simulink model "config5sim_KinematicController_generator"  (R2019b)
settings: Solver=ode4  StartTime=0.0  StopTime=80  FixedStep=0.025  RelTol=1e-3  EnableMultiTasking=on
InitFcn:
  | if set_path == 1
  |     Ref_Path1;
  | elseif set_path == 2
  |     Ref_Path2;
  | elseif set_path == 3
  |     Ref_Path3;
  | end
  | 
  | roboparam;
StopFcn:
  | figure(double(set_path))
  | plot(xyref.DATA(:,1),xyref.DATA(:,2),'--black')
  | hold on
  | plot(xy_axon.DATA(:,1),xy_axon.DATA(:,2),'red')
  | hold on
  | plot(xy_trolley.DATA(:,1),xy_trolley.DATA(:,2),'green')
  | hold on
  | legend('Reference trajectory', 'Robot trajectory', 'Trailer trajectory')
values from neighbouring files (symbols this model uses):
  L = 0.387/2    (= 0.1935)    [AXON_Dynamics_CONF5_vw_old.m]    (also in roboparam.m)
  psicw10 = 0    [roboparam.m]
  psicw20 = 0    [roboparam.m]
  psicw30 = 0    [roboparam.m]
  psicw40 = 0    [roboparam.m]
  rho0 = 0.5    [AXON_Dynamics_CONF5_vw_old.m]    (also in roboparam.m)
  rho1 = 1    [AXON_Dynamics_CONF5_vw_old.m]    (also in roboparam.m)
  rhoH = 0.075    [AXON_Dynamics_CONF5_vw_old.m]    (also in roboparam.m)
  th0 = z(4)    [AXON_Dynamics_CONF5_vw_old.m]    (also in AllInOneDynamic.m = th(i,2); Kinematics.m; PathGenerationPlotting_Dynamics.m = th(i,2); PathGenerationPlotting_Kinematics.m = z(i,4))
  th1 = z(3)    [AXON_Dynamics_CONF5_vw_old.m]    (also in AllInOneDynamic.m = th(i,1); Kinematics.m; PathGenerationPlotting_Dynamics.m = th(i,1); PathGenerationPlotting_Kinematics.m = z(i,3))
  v0 = 0    [roboparam.m]
  w0 = 0    [roboparam.m]
  xaxon0 = xtrolley0+rho1*cos(th1)+rho0*cos(th0)    [roboparam.m]
  xtrolley0 = 0    [roboparam.m]
  yaxon0 = ytrolley0+rho1*sin(th1)+rho0*sin(th0)    [roboparam.m]
  ytrolley0 = 0    [roboparam.m]
undefined symbols (not defined in the file or in its folder): sigbuilder_block
libraries: simulink x2
settings Model: Creator=e0010448  LastModifiedBy=vladkhon
settings DataIOCC: LimitDataPoints=on  SaveFormat=StructureWithTime  ReturnWorkspaceOutputs=off
settings OptimizationCC: BlockReduction=off  BufferReuse=off  LifeSpan=inf
settings DebuggingCC: AlgebraicLoopMsg=none  UnconnectedInputMsg=none  UnconnectedOutputMsg=none  UnconnectedLineMsg=none  AllowSymbolicDim=off  SFUnexpectedBacktrackingDiag=warning  SFNoUnconditionalDefaultTransitionDiag=warning  SFExecutionAtInitializationDiag=none  ArithmeticOperatorsInVariantConditions=warning
settings HardwareCC: ProdBitPerPointer=32  ProdBitPerSizeT=32  ProdBitPerPtrDiffT=32  ProdLargestAtomicFloat=None  ProdIntDivRoundTo=Undefined  ProdEndianess=Unspecified  ProdWordSize=32  ProdHWDeviceType=32-bit Generic
settings ModelReferenceCC: PropagateSignalLabelsOutOfModel=off
settings SFSimCC: SimUseLocalCustomCode=off  CustomCodeUndefinedFunction=UseInterfaceOnly
settings RTWCC: RTWUseLocalCustomCode=off
settings CodeAppCC: StateflowObjectComments=on
settings GRTTargetCC: TargetLangStandard=C89/C90 (ANSI)  GeneratePreprocessorConditionals=Disable all
settings ConfigComp: CovMetricSettings=dw  CovHtmlReporting=on  CovSaveCumulativeToWorkspaceVar=on  CovSaveSingleToWorkspaceVar=on  CovExternalEMLEnable=off

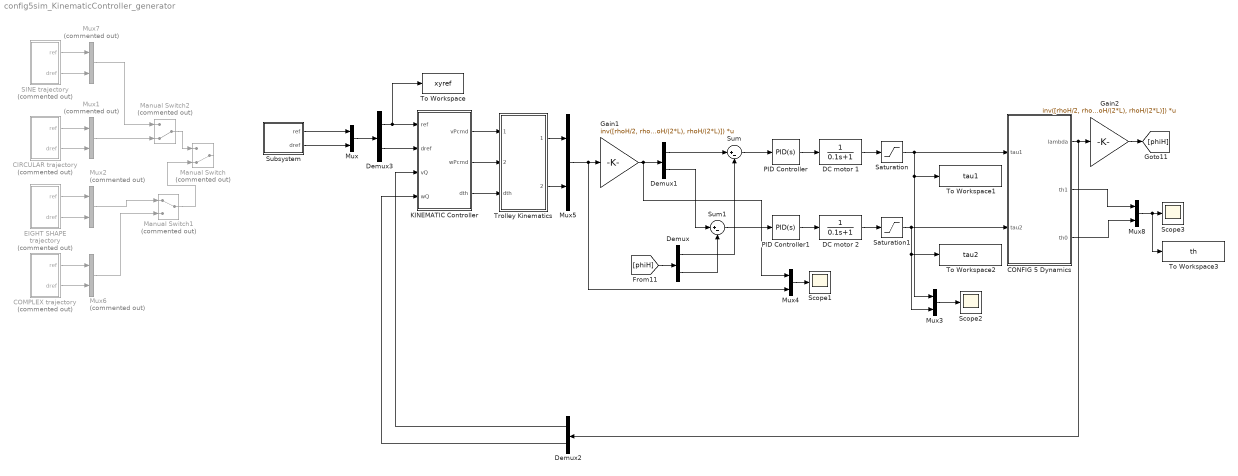
== system config5sim_KinematicController_generator ==
  CIRCULAR trajectory : Subsystem  Commented=on
  COMPLEX trajectory : Subsystem  Commented=on
  CONFIG 5 Dynamics : Subsystem
  DC motor 1 : TransferFcn  Denominator=[0.1 1]
  DC motor 2 : TransferFcn  Denominator=[0.1 1]
  Demux{,1..3} (4 alike) : Demux  Outputs=2
  EIGHT SHAPE trajectory : Subsystem  Commented=on
  Gain1 : Gain  Gain=inv([rhoH/2, rhoH/2; -rhoH/(2*L), rhoH/(2*L)])  Multiplication=Matrix(K*u)
  Gain2 : Gain  Gain=inv([rhoH/2, rhoH/2; -rhoH/(2*L), rhoH/(2*L)])  Multiplication=Matrix(K*u)
  KINEMATIC Controller : Subsystem
  Manual Switch : ManualSwitch  Commented=on  CurrentSetting=0
  Manual Switch1 : ManualSwitch  Commented=on
  Manual Switch2 : ManualSwitch  Commented=on  CurrentSetting=0
  Mux{,3..5,8} (5 alike) : Mux  Inputs=2
  Mux{1..2,6..7} (4 alike) : Mux  Commented=on  Inputs=2
  PID Controller : simulink/Continuous/PID Controller  Controller=PID  Form=Parallel  TimeDomain=Continuous-time  SampleTime=-1  IntegratorMethod=Forward Euler  FilterMethod=Forward Euler  ControllerParametersSource=internal  P=3  I=5  D=1  UseFilter=on  N=100  TunerSelectOption=Transfer Function Based (PID Tuner App)  InitialConditionSource=internal  InitialConditionForIntegrator=0  InitialConditionForFilter=0  DifferentiatorICPrevScaledInput=0  ExternalReset=none  TrackingMode=off  Kt=1  LimitOutput=off  UpperSaturationLimit=inf  LowerSaturationLimit=-inf  LinearizeAsGain=on  AntiWindupMode=none  Kb=1  POutMin=[]  POutMax=[]  IOutMin=[]  IOutMax=[]  DOutMin=[]  DOutMax=[]  NOutMin=[]  NOutMax=[]  SumOutMin=[]  SumOutMax=[]  SaturationOutMin=[]  SaturationOutMax=[]  PParamMin=[]  PParamMax=[]  IParamMin=[]  IParamMax=[]  DParamMin=[]  DParamMax=[]  NParamMin=[]  NParamMax=[]  KbParamMin=[]  KbParamMax=[]  KtParamMin=[]  KtParamMax=[]  KbOutMin=[]  KbOutMax=[]  KtOutMin=[]  KtOutMax=[]  IntegratorOutMin=[]  IntegratorOutMax=[]  FilterOutMin=[]  FilterOutMax=[]  SumI1OutMin=[]  SumI1OutMax=[]  SumI2OutMin=[]  SumI2OutMax=[]  SumI3OutMin=[]  SumI3OutMax=[]  SumI4OutMin=[]  SumI4OutMax=[]  SumDOutMin=[]  SumDOutMax=[]  DifferentiatorOutMin=[]  DifferentiatorOutMax=[]  FilterDiffOutCoefMin=[]  FilterDiffOutCoefMax=[]  ReciprocalOutMin=[]  ReciprocalOutMax=[]  SumDenOutMin=[]  SumDenOutMax=[]  SumNumOutMin=[]  SumNumOutMax=[]  DivideOutMin=[]  DivideOutMax=[]  IntegratorContinuousStateAttributes=''  IntegratorStateMustResolveToSignalObject=off  IntegratorRTWStateStorageClass=Auto  FilterContinuousStateAttributes=''  FilterStateMustResolveToSignalObject=off  FilterRTWStateStorageClass=Auto  ParallelPVariant=InternalParameters  IdealPVariant=Disabled  IVariant=InternalParameters  DVariant=InternalParameters  IntegratorVariant=Continuous  SatVariant=Disabled  AWVariant=Passthrough  PCopyVariant=Disabled  TRVariant=Disabled  FdbkBlocksVariant=Forward  IdealPFdbkVariant=Disabled  SatFdbkVariant=Disabled  DerivativeFilterVariant=ContFilter  NVariant=InternalParameters  NCopyVariant=Disabled  FilterICVariant=InternalICsFilter  IntegratorICVariant=InternalICs  ExternalResetVariant=Disabled  TRSumVariant=Passthrough  SumFdbkVariant=Disabled  SumVariant=Sum_PID
  PID Controller1 : simulink/Continuous/PID Controller  Controller=PID  Form=Parallel  TimeDomain=Continuous-time  SampleTime=-1  IntegratorMethod=Forward Euler  FilterMethod=Forward Euler  ControllerParametersSource=internal  P=3  I=5  D=1  UseFilter=on  N=100  TunerSelectOption=Transfer Function Based (PID Tuner App)  InitialConditionSource=internal  InitialConditionForIntegrator=0  InitialConditionForFilter=0  DifferentiatorICPrevScaledInput=0  ExternalReset=none  TrackingMode=off  Kt=1  LimitOutput=off  UpperSaturationLimit=inf  LowerSaturationLimit=-inf  LinearizeAsGain=on  AntiWindupMode=none  Kb=1  POutMin=[]  POutMax=[]  IOutMin=[]  IOutMax=[]  DOutMin=[]  DOutMax=[]  NOutMin=[]  NOutMax=[]  SumOutMin=[]  SumOutMax=[]  SaturationOutMin=[]  SaturationOutMax=[]  PParamMin=[]  PParamMax=[]  IParamMin=[]  IParamMax=[]  DParamMin=[]  DParamMax=[]  NParamMin=[]  NParamMax=[]  KbParamMin=[]  KbParamMax=[]  KtParamMin=[]  KtParamMax=[]  KbOutMin=[]  KbOutMax=[]  KtOutMin=[]  KtOutMax=[]  IntegratorOutMin=[]  IntegratorOutMax=[]  FilterOutMin=[]  FilterOutMax=[]  SumI1OutMin=[]  SumI1OutMax=[]  SumI2OutMin=[]  SumI2OutMax=[]  SumI3OutMin=[]  SumI3OutMax=[]  SumI4OutMin=[]  SumI4OutMax=[]  SumDOutMin=[]  SumDOutMax=[]  DifferentiatorOutMin=[]  DifferentiatorOutMax=[]  FilterDiffOutCoefMin=[]  FilterDiffOutCoefMax=[]  ReciprocalOutMin=[]  ReciprocalOutMax=[]  SumDenOutMin=[]  SumDenOutMax=[]  SumNumOutMin=[]  SumNumOutMax=[]  DivideOutMin=[]  DivideOutMax=[]  IntegratorContinuousStateAttributes=''  IntegratorStateMustResolveToSignalObject=off  IntegratorRTWStateStorageClass=Auto  FilterContinuousStateAttributes=''  FilterStateMustResolveToSignalObject=off  FilterRTWStateStorageClass=Auto  ParallelPVariant=InternalParameters  IdealPVariant=Disabled  IVariant=InternalParameters  DVariant=InternalParameters  IntegratorVariant=Continuous  SatVariant=Disabled  AWVariant=Passthrough  PCopyVariant=Disabled  TRVariant=Disabled  FdbkBlocksVariant=Forward  IdealPFdbkVariant=Disabled  SatFdbkVariant=Disabled  DerivativeFilterVariant=ContFilter  NVariant=InternalParameters  NCopyVariant=Disabled  FilterICVariant=InternalICsFilter  IntegratorICVariant=InternalICs  ExternalResetVariant=Disabled  TRSumVariant=Passthrough  SumFdbkVariant=Disabled  SumVariant=Sum_PID
  SINE trajectory : Subsystem  Commented=on
  Saturation : Saturate  UpperLimit=40  LowerLimit=-40
  Saturation1 : Saturate  UpperLimit=40  LowerLimit=-40
  Scope1 : Scope
  Scope2 : Scope
  Scope3 : Scope
  Subsystem : Subsystem
  Sum : Sum  Inputs=|+-
  Sum1 : Sum  Inputs=|+-
  To Workspace : ToWorkspace  VariableName=xyref  SaveFormat=Timeseries  SampleTime=-1
  To Workspace1 : ToWorkspace  VariableName=tau1  SampleTime=-1
  To Workspace2 : ToWorkspace  VariableName=tau2  SampleTime=-1
  To Workspace3 : ToWorkspace  VariableName=th  SampleTime=-1
  Trolley Kinematics : Subsystem
  wires:
  Sum/1 -> PID Controller/1
  CONFIG 5 Dynamics/1(lambda) -> Gain2/1, Demux2/1
  [phiH] -> Demux/1
  Demux/1 -> Sum/2
  Demux/2 -> Sum1/2
  Sum1/1 -> PID Controller1/1
  Mux4/1 -> Scope1/1
  Mux5/1 -> Mux4/2, Gain1/1
  Gain2/1 -> [phiH]
  Demux1/1 -> Sum/1
  Demux1/2 -> Sum1/1
  Mux3/1 -> Scope2/1
  Gain1/1 -> Mux4/1, Demux1/1
  PID Controller/1 -> DC motor 1/1
  PID Controller1/1 -> DC motor 2/1
  Demux2/1 -> KINEMATIC Controller/3(vQ)
  Demux2/2 -> KINEMATIC Controller/4(wQ)
  CIRCULAR trajectory/1(ref) -> Mux1/1
  CIRCULAR trajectory/2(dref) -> Mux1/2
  Demux3/1 -> To Workspace/1, KINEMATIC Controller/1(ref)
  Demux3/2 -> KINEMATIC Controller/2(dref)
  EIGHT SHAPE trajectory/1(ref) -> Mux2/1
  EIGHT SHAPE trajectory/2(dref) -> Mux2/2
  Mux2/1 -> Manual Switch1/1
  Manual Switch1/1 -> Manual Switch/2
  Mux6/1 -> Manual Switch1/2
  COMPLEX trajectory/1(ref) -> Mux6/1
  COMPLEX trajectory/2(dref) -> Mux6/2
  Manual Switch2/1 -> Manual Switch/1
  Mux1/1 -> Manual Switch2/2
  Mux7/1 -> Manual Switch2/1
  SINE trajectory/1(ref) -> Mux7/1
  SINE trajectory/2(dref) -> Mux7/2
  DC motor 1/1 -> Saturation/1
  Saturation/1 -> To Workspace1/1, Mux3/1, CONFIG 5 Dynamics/1(tau1)
  DC motor 2/1 -> Saturation1/1
  Saturation1/1 -> To Workspace2/1, Mux3/2, CONFIG 5 Dynamics/2(tau2)
  KINEMATIC Controller/1(vPcmd) -> Trolley Kinematics/1(vPcmd)
  KINEMATIC Controller/2(wPcmd) -> Trolley Kinematics/2(wPcmd)
  Trolley Kinematics/1(vQcmd) -> Mux5/1
  Trolley Kinematics/2(wQcmd) -> Mux5/2
  KINEMATIC Controller/3(dth) -> Trolley Kinematics/3(dth)
  Mux8/1 -> To Workspace3/1, Scope3/1
  Subsystem/2("dref ") -> Mux/2
  Subsystem/1(ref) -> Mux/1
  Mux/1 -> Demux3/1
  CONFIG 5 Dynamics/3(th0) -> Mux8/2
  CONFIG 5 Dynamics/2(th1) -> Mux8/1

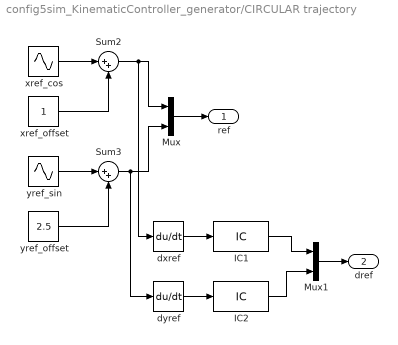
== system config5sim_KinematicController_generator/CIRCULAR trajectory ==
  IC1 : InitialCondition  Value=0
  IC2 : InitialCondition  Value=7.5*0.05
  Mux : Mux  Inputs=2
  Mux1 : Mux  Inputs=2
  Sum2 : Sum  Inputs=|++
  Sum3 : Sum  Inputs=|++
  dxref : Derivative  CoefficientInTFapproximation=100
  dyref : Derivative  CoefficientInTFapproximation=100
  xref_cos : Sin  Amplitude=25  Frequency=0.05  Phase=pi/2  Samples=100  SampleTime=0  Offset=10
  xref_offset : Constant
  yref_offset : Constant  Value=2.5
  yref_sin : Sin  Amplitude=25  Frequency=0.05  Samples=100  SampleTime=0  Offset=10
  ref : Outport  VectorParamsAs1DForOutWhenUnconnected=off
  dref : Outport  Port=2  VectorParamsAs1DForOutWhenUnconnected=off
  wires:
  xref_cos/1 -> Sum2/1
  yref_sin/1 -> Sum3/1
  xref_offset/1 -> Sum2/2
  Sum2/1 -> dxref/1, Mux/1
  yref_offset/1 -> Sum3/2
  Sum3/1 -> dyref/1, Mux/2
  Mux/1 -> ref/1
  dxref/1 -> IC1/1
  dyref/1 -> IC2/1
  IC2/1 -> Mux1/2
  IC1/1 -> Mux1/1
  Mux1/1 -> dref/1

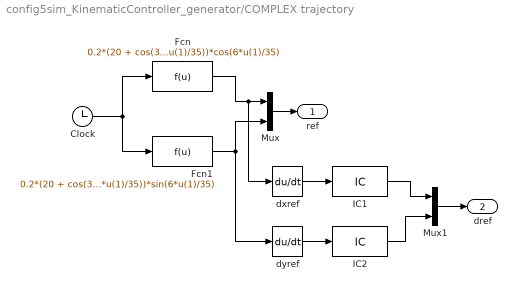
== system config5sim_KinematicController_generator/COMPLEX trajectory ==
  Clock : Clock
  Fcn : Fcn  Expr=0.2*(20 + cos(36*u(1)/35))*cos(6*u(1)/35)
  Fcn1 : Fcn  Expr=0.2*(20 + cos(36*u(1)/35))*sin(6*u(1)/35)
  IC1 : InitialCondition  Value=0
  IC2 : InitialCondition  Value=18*0.2/5
  Mux : Mux  Inputs=2
  Mux1 : Mux  Inputs=2
  dxref : Derivative  CoefficientInTFapproximation=100
  dyref : Derivative  CoefficientInTFapproximation=100
  ref : Outport  VectorParamsAs1DForOutWhenUnconnected=off
  dref : Outport  Port=2  VectorParamsAs1DForOutWhenUnconnected=off
  wires:
  Clock/1 -> Fcn1/1, Fcn/1
  Mux/1 -> ref/1
  dxref/1 -> IC1/1
  dyref/1 -> IC2/1
  IC2/1 -> Mux1/2
  IC1/1 -> Mux1/1
  Mux1/1 -> dref/1
  Fcn/1 -> dxref/1, Mux/1
  Fcn1/1 -> dyref/1, Mux/2

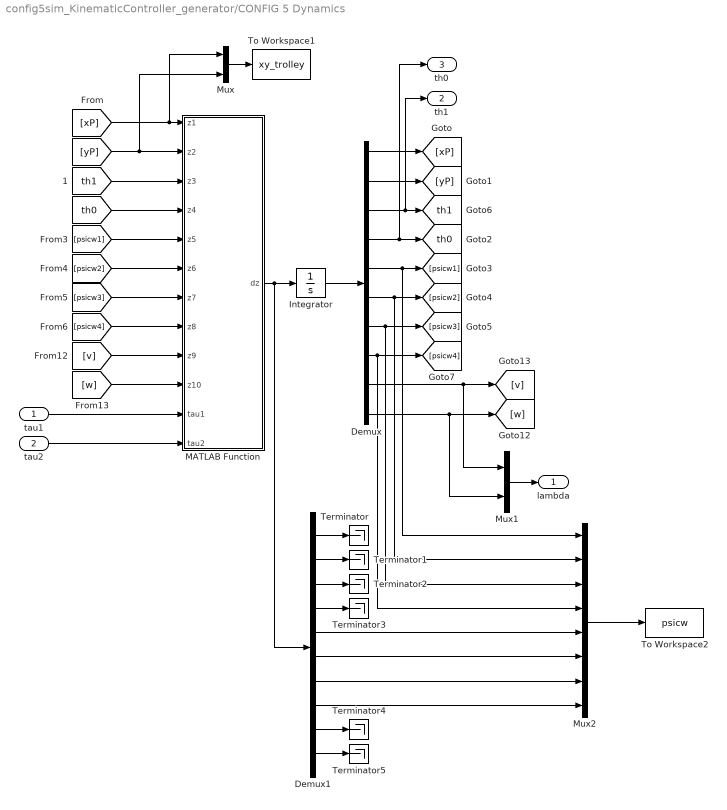
== system config5sim_KinematicController_generator/CONFIG 5 Dynamics ==
  tau1 : Inport
  tau2 : Inport  Port=2
  Demux : Demux  Outputs=10
  Demux1 : Demux  Outputs=10
  Integrator : Integrator  InitialCondition=[xtrolley0 ytrolley0 th1 th0 psicw10 psicw20 psicw30 psicw40 v0 w0]
  MATLAB Function : MATLAB Function  TreatAsAtomicUnit=on
  Mux : Mux  Inputs=2
  Mux1 : Mux  Inputs=2
  Mux2 : Mux  Inputs=8
  Terminator{,1..5} (6 alike) : Terminator
  To Workspace1 : ToWorkspace  VariableName=xy_trolley  SaveFormat=Timeseries  SampleTime=-1
  To Workspace2 : ToWorkspace  VariableName=psicw  SaveFormat=Timeseries  SampleTime=-1
  lambda : Outport  VectorParamsAs1DForOutWhenUnconnected=off
  th1 : Outport  Port=2  VectorParamsAs1DForOutWhenUnconnected=off
  th0 : Outport  Port=3  VectorParamsAs1DForOutWhenUnconnected=off
  tag scope: th0=global, th1=global
  wires:
  Mux1/1 -> lambda/1
  Integrator/1 -> Demux/1
  Demux/10 -> Mux1/2, [w]
  Demux/9 -> Mux1/1, [v]
  Demux/8 -> [psicw4], Mux2/4
  Demux/7 -> [psicw3], Mux2/3
  Demux/6 -> [psicw2], Mux2/2
  Demux/5 -> [psicw1], Mux2/1
  Demux/2 -> [yP]
  Demux/1 -> [xP]
  MATLAB Function/1(dz) -> Demux1/1, Integrator/1
  [xP] -> Mux/1, MATLAB Function/1(z1)
  [yP] -> Mux/2, MATLAB Function/2(z2)
  [psicw1] -> MATLAB Function/5(z5)
  [psicw2] -> MATLAB Function/6(z6)
  [psicw3] -> MATLAB Function/7(z7)
  [psicw4] -> MATLAB Function/8(z8)
  [v] -> MATLAB Function/9(z9)
  [w] -> MATLAB Function/10(z10)
  [th1] -> MATLAB Function/3(z3)
  [th0] -> MATLAB Function/4(z4)
  Demux/3 -> th1/1, [th1]
  Demux/4 -> th0/1, [th0]
  tau1/1 -> MATLAB Function/11(tau1)
  tau2/1 -> MATLAB Function/12(tau2)
  Demux1/8 -> Mux2/8
  Demux1/7 -> Mux2/7
  Demux1/6 -> Mux2/6
  Demux1/5 -> Mux2/5
  Mux2/1 -> To Workspace2/1
  Demux1/1 -> Terminator/1
  Demux1/2 -> Terminator1/1
  Demux1/4 -> Terminator3/1
  Demux1/3 -> Terminator2/1
  Demux1/10 -> Terminator5/1
  Demux1/9 -> Terminator4/1
  Mux/1 -> To Workspace1/1

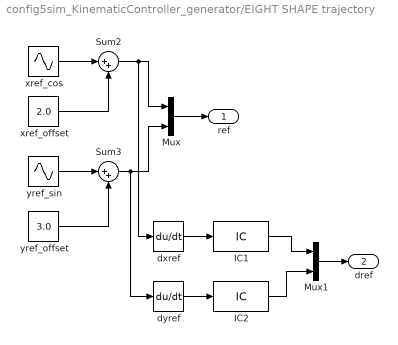
== system config5sim_KinematicController_generator/EIGHT SHAPE trajectory ==
  IC1 : InitialCondition  Value=2*0.1
  IC2 : InitialCondition  Value=2*0.05
  Mux : Mux  Inputs=2
  Mux1 : Mux  Inputs=2
  Sum2 : Sum  Inputs=|++
  Sum3 : Sum  Inputs=|++
  dxref : Derivative  CoefficientInTFapproximation=100
  dyref : Derivative  CoefficientInTFapproximation=100
  xref_cos : Sin  Amplitude=2  Frequency=0.1  Samples=100  SampleTime=0  Offset=10
  xref_offset : Constant  Value=2.0
  yref_offset : Constant  Value=3.0
  yref_sin : Sin  Amplitude=2  Frequency=0.05  Samples=100  SampleTime=0  Offset=10
  ref : Outport  VectorParamsAs1DForOutWhenUnconnected=off
  dref : Outport  Port=2  VectorParamsAs1DForOutWhenUnconnected=off
  wires:
  xref_cos/1 -> Sum2/1
  yref_sin/1 -> Sum3/1
  xref_offset/1 -> Sum2/2
  yref_offset/1 -> Sum3/2
  Sum2/1 -> dxref/1, Mux/1
  Sum3/1 -> dyref/1, Mux/2
  Mux/1 -> ref/1
  dxref/1 -> IC1/1
  dyref/1 -> IC2/1
  IC2/1 -> Mux1/2
  IC1/1 -> Mux1/1
  Mux1/1 -> dref/1

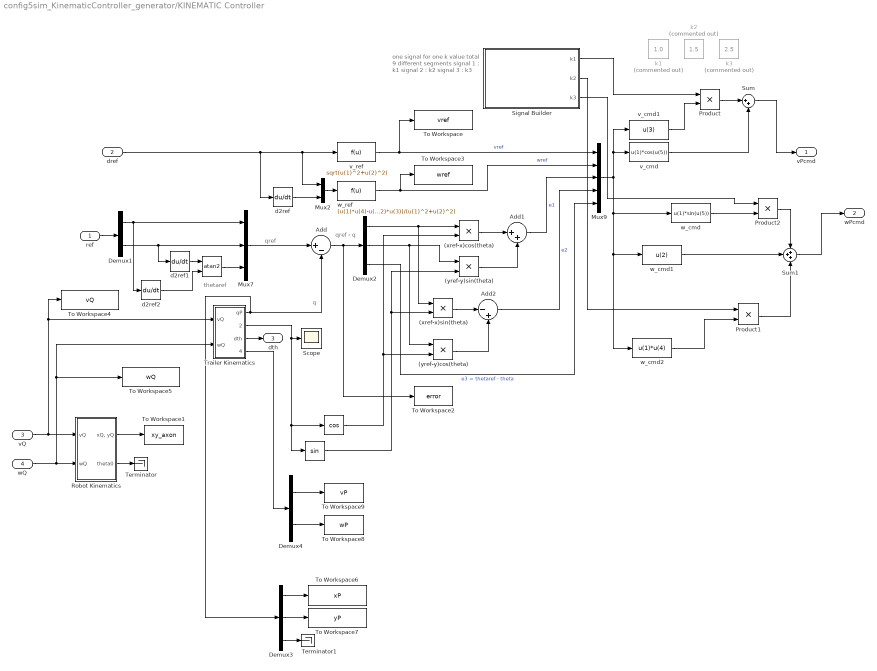
== system config5sim_KinematicController_generator/KINEMATIC Controller ==
  note: one signal for one k value
      | total 9 different segments
      |
      | signal 1 : k1
      | signal 2 : k2
      | signal 3 : k3
  note: qref - q
  note: q
  note: qref
  note: thetaref
  ref : Inport
  dref : Inport  Port=2
  vQ : Inport  Port=3
  wQ : Inport  Port=4
  "     " : Trigonometry  Operator=atan2
  "         " : Trigonometry  Operator=cos
  "          " : Trigonometry
  (xref-x)cos(theta) : Product
  (xref-x)sin(theta) : Product
  (yref-y)cos(theta) : Product
  (yref-y)sin(theta) : Product
  Add : Sum  Inputs=|+-
  Add1 : Sum  Inputs=|++
  Add2 : Sum  Inputs=|-+
  Demux1 : Demux  Outputs=2
  Demux2 : Demux  Outputs=3
  Demux3 : Demux  Outputs=3
  Demux4 : Demux  Outputs=2
  Mux2 : Mux  Inputs=2
  Mux7 : Mux  Inputs=3
  Mux9 : Mux  Inputs=5
  Product : Product
  Product1 : Product
  Product2 : Product
  Robot Kinematics : Subsystem
  Scope : Scope
  Signal Builder : Subsystem  Tag=STV Subsys  LoadFcn=sigbuilder_block('load');  StartFcn=sigbuilder_block('start');  StopFcn=sigbuilder_block('stop');  ClipboardFcn=sigbuilder_block('clipboard');  mask(Sigbuilder block){tuvar=[0:10]}
      mask help: Simulink:masks:SigbuilderBlock_MD
      mask init:
      | if ~strcmp(get_param(bdroot(gcbh),'SimulationStatus'),'stopped') tuvar = sigbuilder_block('maskInit'); end
      settings: CopyFcn=sigbuilder_block('copy');  DeleteFcn=sigbuilder_block('delete');  ModelCloseFcn=sigbuilder_block('modelClose');  PreSaveFcn=sigbuilder_block('preSave');  PauseFcn=sigbuilder_block('pause');  ContinueFcn=sigbuilder_block('continue');  NameChangeFcn=sigbuilder_block('namechange');  OpenFcn=sigbuilder_block('open',[5.5 30 949 418 ]);  CloseFcn=sigbuilder_block('close');
      mask Display: plot(0, 0, 100, 100,[2, 2, 32, 32, 2], [68, 8, 8, 68, 68],[32, 2], [38, 38], [32, 19, 2],[53, 60, 44], [32, 17, 17, 2],[16, 16, 31, 31]);txt = getActiveGroup(gcbh);text(2, 100, txt,'verticalAlignment', 'top');
  Sum : Sum  Inputs=|++
  Sum1 : Sum  Inputs=+++
  Terminator : Terminator
  Terminator1 : Terminator
  To Workspace : ToWorkspace  VariableName=vref  SampleTime=-1
  To Workspace1 : ToWorkspace  VariableName=xy_axon  SaveFormat=Timeseries  SampleTime=-1
  To Workspace2 : ToWorkspace  VariableName=error  SaveFormat=Timeseries  SampleTime=-1
  To Workspace3 : ToWorkspace  VariableName=wref  SampleTime=-1
  To Workspace4 : ToWorkspace  VariableName=vQ  SampleTime=-1
  To Workspace5 : ToWorkspace  VariableName=wQ  SampleTime=-1
  To Workspace6 : ToWorkspace  VariableName=xP  SampleTime=-1
  To Workspace7 : ToWorkspace  VariableName=yP  SampleTime=-1
  To Workspace8 : ToWorkspace  VariableName=wP  SampleTime=-1
  To Workspace9 : ToWorkspace  VariableName=vP  SampleTime=-1
  Trailer Kinematics : Subsystem
  d2ref : Derivative  CoefficientInTFapproximation=100
  d2ref1 : Derivative  CoefficientInTFapproximation=100
  d2ref2 : Derivative  CoefficientInTFapproximation=100
  "k1 " : Constant  Commented=on  Value=1.0
  "k2 " : Constant  Commented=on  Value=1.5
  "k3 " : Constant  Commented=on  Value=2.5
  v_cmd : Fcn  Expr=u(1)*cos(u(5))
  v_cmd1 : Fcn  Expr=u(3)
  v_ref : Fcn  Expr=sqrt(u(1)^2+u(2)^2)
  w_cmd : Fcn  Expr=u(1)*sin(u(5))
  w_cmd1 : Fcn  Expr=u(2)
  w_cmd2 : Fcn  Expr=u(1)*u(4)
  w_ref : Fcn  Expr=(u(1)*u(4)-u(2)*u(3))/(u(1)^2+u(2)^2)
  vPcmd : Outport  VectorParamsAs1DForOutWhenUnconnected=off
  wPcmd : Outport  Port=2  VectorParamsAs1DForOutWhenUnconnected=off
  dth : Outport  Port=3  VectorParamsAs1DForOutWhenUnconnected=off
  wires:
  (xref-x)sin(theta)/1 -> Add2/1
  (yref-y)cos(theta)/1 -> Add2/2
  v_ref/1 -> To Workspace/1, Mux9/1  "vref"
  w_ref/1 -> To Workspace3/1, Mux9/2  "wref"
  Add/1 -> To Workspace2/1, Demux2/1
  Mux2/1 -> w_ref/1
  dref/1 -> d2ref/1, Mux2/1, v_ref/1
  d2ref/1 -> Mux2/2
  Mux7/1 -> Add/1
  Demux2/1 -> (xref-x)sin(theta)/1, (xref-x)cos(theta)/1
  (xref-x)cos(theta)/1 -> Add1/1
  (yref-y)sin(theta)/1 -> Add1/2
  Add1/1 -> Mux9/3  "e1"
  Add2/1 -> Mux9/4  "e2"
  Demux2/3 -> Mux9/5  "e3 = thetaref - theta"
  Demux2/2 -> (yref-y)cos(theta)/1, (yref-y)sin(theta)/1
  "         "/1 -> (yref-y)cos(theta)/2, (xref-x)cos(theta)/2
  "          "/1 -> (xref-x)sin(theta)/2, (yref-y)sin(theta)/2
  Mux9/1 -> w_cmd/1, w_cmd2/1, w_cmd1/1, v_cmd1/1, v_cmd/1
  ref/1 -> Demux1/1
  Demux1/1 -> Mux7/1, d2ref2/1
  Demux1/2 -> d2ref1/1, Mux7/2
  "     "/1 -> Mux7/3
  vQ/1 -> To Workspace4/1, Trailer Kinematics/1(vQ), Robot Kinematics/1(vQ)
  wQ/1 -> Trailer Kinematics/2(wQ), To Workspace5/1, Robot Kinematics/2(wQ)
  Robot Kinematics/1("xQ, yQ") -> To Workspace1/1
  Trailer Kinematics/1(qP) -> Demux3/1, Add/2
  Trailer Kinematics/3(dth) -> dth/1
  Trailer Kinematics/2(theta1) -> "         "/1, "          "/1, Scope/1
  d2ref1/1 -> "     "/1
  d2ref2/1 -> "     "/2
  Robot Kinematics/2(theta0) -> Terminator/1
  v_cmd1/1 -> Product/2
  Product/1 -> Sum/1
  v_cmd/1 -> Sum/2
  Sum/1 -> vPcmd/1
  w_cmd2/1 -> Product1/2
  Sum1/1 -> wPcmd/1
  w_cmd1/1 -> Sum1/2
  Product1/1 -> Sum1/3
  w_cmd/1 -> Product2/2
  Product2/1 -> Sum1/1
  Signal Builder/1(k1) -> Product/1
  Signal Builder/2(k2) -> Product1/1
  Signal Builder/3(k3) -> Product2/1
  Demux3/1 -> To Workspace6/1
  Demux3/2 -> To Workspace7/1
  Demux3/3 -> Terminator1/1
  Demux4/1 -> To Workspace9/1
  Demux4/2 -> To Workspace8/1
  Trailer Kinematics/4("vP, wP") -> Demux4/1

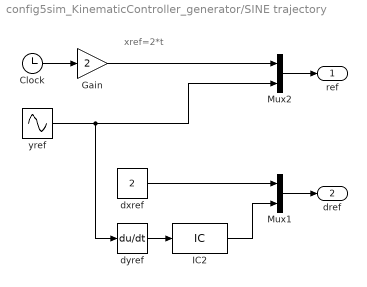
== system config5sim_KinematicController_generator/SINE trajectory ==
  note: xref=2*t
  Clock : Clock
  Gain : Gain  Gain=2
  IC2 : InitialCondition  Value=2*0.25
  Mux1 : Mux  Inputs=2
  Mux2 : Mux  Inputs=2
  dxref : Constant  Value=2
  dyref : Derivative  CoefficientInTFapproximation=100
  yref : Sin  Amplitude=2  Frequency=0.25  Samples=100  SampleTime=0  Offset=10
  ref : Outport  VectorParamsAs1DForOutWhenUnconnected=off
  dref : Outport  Port=2  VectorParamsAs1DForOutWhenUnconnected=off
  wires:
  yref/1 -> Mux2/2, dyref/1
  dyref/1 -> IC2/1
  IC2/1 -> Mux1/2
  dxref/1 -> Mux1/1
  Mux1/1 -> dref/1
  Mux2/1 -> ref/1
  Gain/1 -> Mux2/1
  Clock/1 -> Gain/1

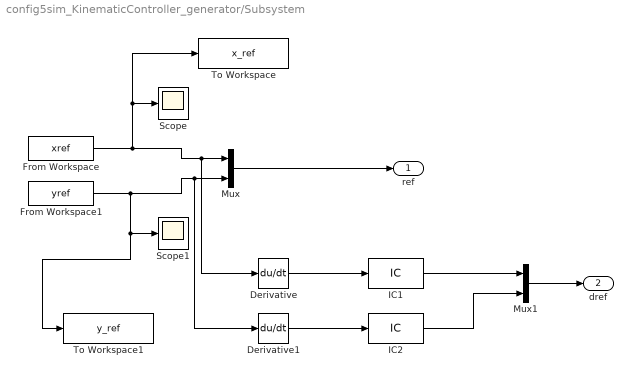
== system config5sim_KinematicController_generator/Subsystem ==
  Derivative : Derivative
  Derivative1 : Derivative
  From Workspace : FromWorkspace  VariableName=xref  SampleTime=0
  From Workspace1 : FromWorkspace  VariableName=yref  SampleTime=0
  IC1 : InitialCondition  Value=0
  IC2 : InitialCondition  Value=0.0001
  Mux : Mux  Inputs=2
  Mux1 : Mux  Inputs=2
  Scope : Scope
  Scope1 : Scope
  To Workspace : ToWorkspace  VariableName=x_ref  SampleTime=-1
  To Workspace1 : ToWorkspace  VariableName=y_ref  SampleTime=-1
  ref : Outport  VectorParamsAs1DForOutWhenUnconnected=off
  "dref " : Outport  Port=2  VectorParamsAs1DForOutWhenUnconnected=off
  wires:
  Mux/1 -> ref/1
  From Workspace/1 -> Derivative/1, Mux/1, Scope/1, To Workspace/1
  From Workspace1/1 -> Derivative1/1, Mux/2, Scope1/1, To Workspace1/1
  Mux1/1 -> "dref "/1
  Derivative/1 -> IC1/1
  Derivative1/1 -> IC2/1
  IC1/1 -> Mux1/1
  IC2/1 -> Mux1/2

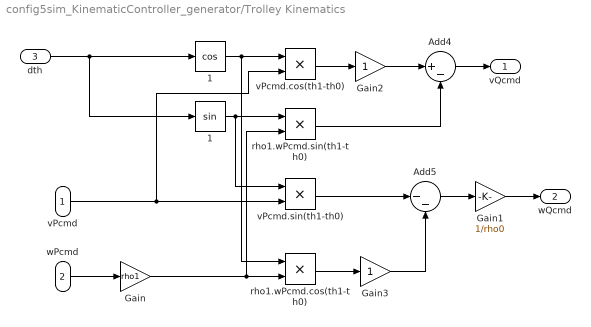
== system config5sim_KinematicController_generator/Trolley Kinematics ==
  vPcmd : Inport
  wPcmd : Inport  Port=2
  dth : Inport  Port=3
  "          1" : Trigonometry
  "         1" : Trigonometry  Operator=cos
  Add4 : Sum  Inputs=|+-
  Add5 : Sum  Inputs=|--
  Gain : Gain  Gain=rho1
  Gain1 : Gain  Gain=1/rho0
  Gain2 : Gain
  Gain3 : Gain
  rho1.wPcmd.cos(th1-th0) : Product
  rho1.wPcmd.sin(th1-th0) : Product
  vPcmd.cos(th1-th0) : Product
  vPcmd.sin(th1-th0) : Product
  vQcmd : Outport  VectorParamsAs1DForOutWhenUnconnected=off
  wQcmd : Outport  Port=2  VectorParamsAs1DForOutWhenUnconnected=off
  wires:
  "         1"/1 -> rho1.wPcmd.cos(th1-th0)/1, vPcmd.cos(th1-th0)/1
  dth/1 -> "         1"/1, "          1"/1
  "          1"/1 -> vPcmd.sin(th1-th0)/1, rho1.wPcmd.sin(th1-th0)/1
  Gain/1 -> rho1.wPcmd.sin(th1-th0)/2, rho1.wPcmd.cos(th1-th0)/2
  rho1.wPcmd.sin(th1-th0)/1 -> Add4/2
  vPcmd/1 -> vPcmd.cos(th1-th0)/2, vPcmd.sin(th1-th0)/2
  wPcmd/1 -> Gain/1
  Add5/1 -> Gain1/1
  Gain1/1 -> wQcmd/1
  vPcmd.sin(th1-th0)/1 -> Add5/1
  Add4/1 -> vQcmd/1
  vPcmd.cos(th1-th0)/1 -> Gain2/1
  Gain2/1 -> Add4/1
  rho1.wPcmd.cos(th1-th0)/1 -> Gain3/1
  Gain3/1 -> Add5/2

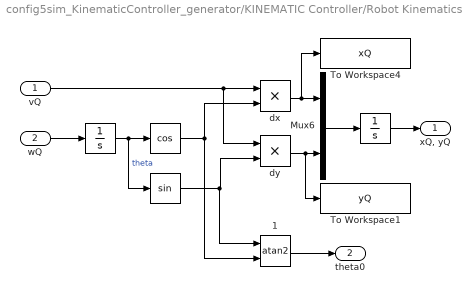
== system config5sim_KinematicController_generator/KINEMATIC Controller/Robot Kinematics ==
  vQ : Inport
  wQ : Inport  Port=2
  " " : Trigonometry  Operator=cos
  "  " : Trigonometry
  "   " : Integrator  InitialCondition=th0
  "    " : Integrator  InitialCondition=[xaxon0 yaxon0]
  "     1" : Trigonometry  Operator=atan2
  Mux6 : Mux  Inputs=2
  To Workspace1 : ToWorkspace  VariableName=yQ  SampleTime=-1
  To Workspace4 : ToWorkspace  VariableName=xQ  SampleTime=-1
  dx : Product
  dy : Product
  "xQ, yQ" : Outport  VectorParamsAs1DForOutWhenUnconnected=off
  theta0 : Outport  Port=2  VectorParamsAs1DForOutWhenUnconnected=off
  wires:
  dx/1 -> To Workspace4/1, Mux6/1
  dy/1 -> To Workspace1/1, Mux6/2
  vQ/1 -> dy/1, dx/1
  wQ/1 -> "   "/1
  " "/1 -> "     1"/2, dx/2
  "   "/1 -> "  "/1, " "/1  "theta"
  "  "/1 -> "     1"/1, dy/2
  Mux6/1 -> "    "/1
  "    "/1 -> "xQ, yQ"/1
  "     1"/1 -> theta0/1

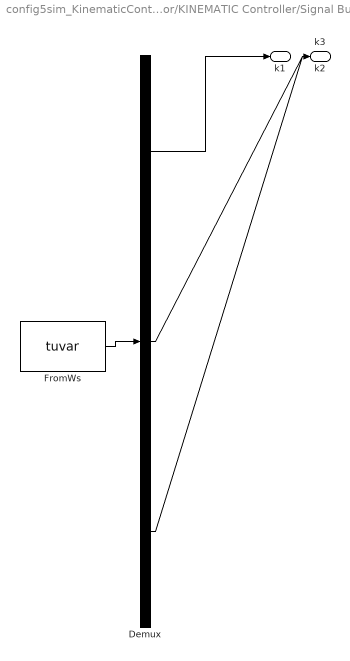
== system config5sim_KinematicController_generator/KINEMATIC Controller/Signal Builder ==
  Demux : Demux  Tag=STV Demux  Outputs=3
  FromWs : FromWorkspace  Tag=STV FromWs  VariableName=tuvar  SampleTime=0
      SigBuilderData=|
      | common.afterFinalStr = 'Extrapolate'
      | common.sampleTime = 0
      | dataSet.timeRange = [0 60]
      | dataSet.name = 'Kinematic control parameters'
      | sbobj.Groups.Name = 'Kinematic control parameters'
      | sbobj.Groups.Signals(1).Name = 'k1'
      | sbobj.Groups.Signals(1).XData = [0 6.5 6.5 13.375 13.375 19.875 19.875 26.75 26.75 33.25 33.25 40.125 40.125 46.625 46.625 53.5 53.5 60]
      | sbobj.Groups.Signals(1).YData = [0.8 0.8 0.6 0.6 0.25 0.25 0.3 0.3 0.8 0.8 0.3 0.3 0.25 0.25 0.6 0.6 0.8 0.8]
      | sbobj.Groups.Signals(2).Name = 'k2'
      | sbobj.Groups.Signals(2).XData = [0 6.5 6.5 13.375 13.375 19.875 19.875 26.7379679144 26.75 33.25 33.25 40.125 40.125 46.625 46.625 53.5 53.5 60]
      | sbobj.Groups.Signals(2).YData = [0.1 0.1 2.8 2.8 1.6 1.6 1.8 1.8 0.1 0.1 1.8 1.8 1.6 1.6 2.8 2.8 0.1 0.1]
      | sbobj.Groups.Signals(3).Name = 'k3'
      | sbobj.Groups.Signals(3).XData = [0 6.5 6.5 13.375 13.375 19.875 19.875 26.75 26.75 33.25 33.25 40.125 40.125 46.625 46.625 53.5 53.5 60]
      | sbobj.Groups.Signals(3).YData = [1.5 1.5 2.5 2.5 2 2 5.1 5.1 1.5 1.5 5.1 5.1 2 2 2.5 2.5 1.5 1.5]
      | sbobj.Groups.TimeRange = [0 60]
  k1 : Outport  Tag=STV Outport  VectorParamsAs1DForOutWhenUnconnected=off
  k2 : Outport  Tag=STV Outport  Port=2  VectorParamsAs1DForOutWhenUnconnected=off
  k3 : Outport  Tag=STV Outport  Port=3  VectorParamsAs1DForOutWhenUnconnected=off
  wires:
  Demux/1 -> k1/1
  FromWs/1 -> Demux/1
  Demux/2 -> k2/1
  Demux/3 -> k3/1

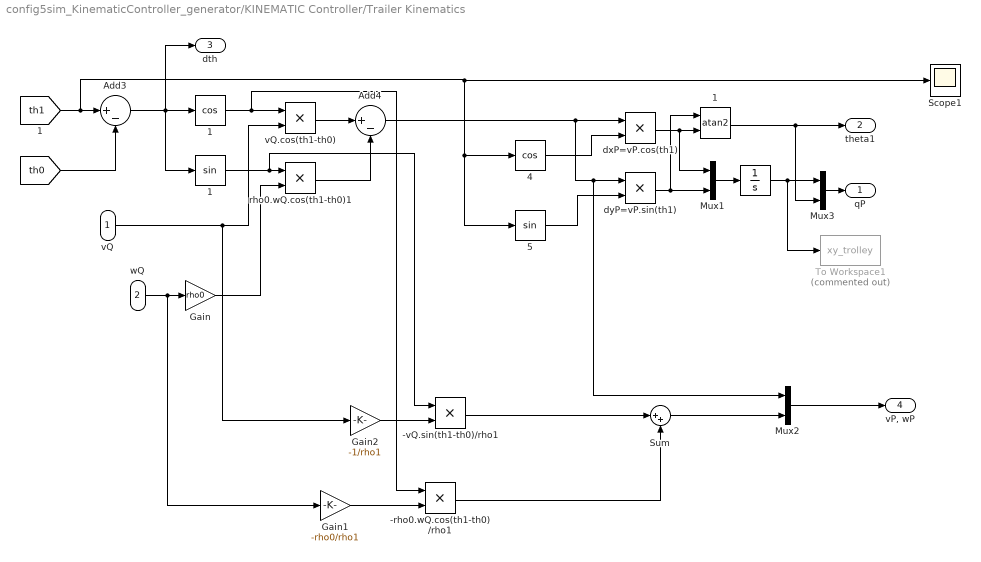
== system config5sim_KinematicController_generator/KINEMATIC Controller/Trailer Kinematics ==
  vQ : Inport
  wQ : Inport  Port=2
  "    " : Integrator  InitialCondition=[xtrolley0 ytrolley0]
  "          1" : Trigonometry
  "         1" : Trigonometry  Operator=cos
  "         4" : Trigonometry  Operator=cos
  "         5" : Trigonometry
  "     1" : Trigonometry  Operator=atan2
  -rho0.wQ.cos(th1-th0)/rho1 : Product
  -vQ.sin(th1-th0)/rho1 : Product
  Add3 : Sum  Inputs=|+-
  Add4 : Sum  Inputs=|+-
  Gain : Gain  Gain=rho0
  Gain1 : Gain  Gain=-rho0/rho1
  Gain2 : Gain  Gain=-1/rho1
  Mux1 : Mux  Inputs=2
  Mux2 : Mux  Inputs=2
  Mux3 : Mux  Inputs=2
  Scope1 : Scope
  Sum : Sum  Inputs=|++
  To Workspace1 : ToWorkspace  Commented=on  VariableName=xy_trolley  SaveFormat=Timeseries  SampleTime=-1
  dxP=vP.cos(th1) : Product
  dyP=vP.sin(th1) : Product
  rho0.wQ.cos(th1-th0)1 : Product
  vQ.cos(th1-th0) : Product
  qP : Outport  VectorParamsAs1DForOutWhenUnconnected=off
  theta1 : Outport  Port=2  VectorParamsAs1DForOutWhenUnconnected=off
  dth : Outport  Port=3  VectorParamsAs1DForOutWhenUnconnected=off
  "vP, wP" : Outport  Port=4  VectorParamsAs1DForOutWhenUnconnected=off
  wires:
  "     1"/1 -> theta1/1, Mux3/2
  "    "/1 -> To Workspace1/1, Mux3/1
  vQ.cos(th1-th0)/1 -> Add4/1
  Add3/1 -> dth/1, "          1"/1, "         1"/1
  Gain/1 -> rho0.wQ.cos(th1-th0)1/2
  dyP=vP.sin(th1)/1 -> Mux1/2, "     1"/1
  rho0.wQ.cos(th1-th0)1/1 -> Add4/2
  Mux3/1 -> qP/1
  Mux1/1 -> "    "/1
  Add4/1 -> Mux2/1, dyP=vP.sin(th1)/1, dxP=vP.cos(th1)/1
  dxP=vP.cos(th1)/1 -> "     1"/2, Mux1/1
  [th1] -> Scope1/1, "         5"/1, "         4"/1, Add3/1
  [th0] -> Add3/2
  "         4"/1 -> dxP=vP.cos(th1)/2
  "         5"/1 -> dyP=vP.sin(th1)/2
  -vQ.sin(th1-th0)/rho1/1 -> Sum/1
  wQ/1 -> Gain1/1, Gain/1
  Gain2/1 -> -vQ.sin(th1-th0)/rho1/2
  Mux2/1 -> "vP, wP"/1
  Sum/1 -> Mux2/2
  Gain1/1 -> -rho0.wQ.cos(th1-th0)/rho1/2
  -rho0.wQ.cos(th1-th0)/rho1/1 -> Sum/2
  vQ/1 -> Gain2/1, vQ.cos(th1-th0)/2
  "         1"/1 -> -rho0.wQ.cos(th1-th0)/rho1/1, vQ.cos(th1-th0)/1
  "          1"/1 -> -vQ.sin(th1-th0)/rho1/1, rho0.wQ.cos(th1-th0)1/1

== matlab function config5sim_KinematicController_generator/CONFIG 5 Dynamics/MATLAB Function ==
  data: z1 input; dz output; z2 input; z3 input; z4 input; z5 input; z6 input; z7 input; z8 input; z9 input; z10 input; tau1 input; tau2 input
function dz = AXON_Dynamics_CONF5_VW_Simulink(z1,z2,z3,z4,z5,z6,z7,z8,z9,z10,tau1,tau2)
%% ODE function for the dynamics of configuration 5 that uses linear and angular velocity states
% t -> time variable
% z -> state variables  [x,y,th1,th0,psicw(4),v,w]

% variable state assignment

% position of pt P (x,y) axon orientation (th0) and trolley orientation (th1)
x = z1;
y = z2;
th1 = z3;
th0 = z4;

% caster wheel orientation (psicw_i)
psicw1 = z5;
psicw2 = z6;
psicw3 = z7;
psicw4 = z8;

% linear and angular velocity of and about point Q (v,w)
v = z9;
w = z10;

% distance in m
rho0 = 0.5;%0.5; 
rho1 = 1;%1;

L = 0.387/2;
s_l = 0.928;
s_w = 0.48;
dcw = 0.075;
dqpx = 0;  % distance bet q and P
dqcmBx = 0*0.648/4; % distance bet Q and Axon Centre of Mass
cw1x = -s_l/2;
cw1_x = cw1x;
cw3x =  s_l/2;
cw3_x = cw3x;
dpcmPx = 0; %s_l/2;

% mass in kg
mB = 50;
m_P = 150;
mH = 2;
mW = 0.7;
mCW = 5.0; 
mT = m_P + 2*mW + 2*mH + 2*mCW +mB;

% wheel radius and distances
rhoH = 0.075;
rho_h = rhoH;
rhow = 0.06;
rho_w = rhow;
rhocw = 0.05;
rho_cw = rhocw;
rho0 = 0.5;     % 0.5; 
rho1 = 1;       % distance in m

e1 = (2*mH + mB)*rho1 + dpcmPx*m_P - 2*mCW*s_l; % dqpx*m_P + 2*mCW*(cw3x + cw1x) + dqcmBx*mB;
e2 = (2*mH + mB)*rho0 + dqcmBx*mB;

IWy = (1/2)*mW*rho_w^2;
IWz = (1/12)*mW*(3*rho_w^2 + 0.03^2);
ICWz = (1/12)*mCW*(3*rho_cw^2 + 0.01^2);
IPz = (1/12)*m_P*(s_l^2 + (2*s_w)^2);
IBz = (1/12)*mB*(0.3^2 + 0.6^2);
IHz = (1/12)*mH*(3*rho_h^2 + 0.03^2);
IHy = (1/2)*mH*rho_h^2;

ITw = IWz + s_w^2*mW;
ITCWz = ICWz + mCW*dcw^2;
ITB = IBz + mB*dqcmBx^2;
ITH = IHz + mH*L^2;
IT_P = IPz + m_P*dpcmPx^2;

ITz = (2*mH + mB)*rho0^2 + 2*dqcmBx*mB*rho0 + ITB + 2*ITH;
ITP = (2*mH + mB)*rho1^2 + IT_P + 2*ITw + 2*mCW*(s_w^2 + s_l^2);

T = rhoH/2*[1, 1; -1/L 1/L]; % transformation matrix for driving wheels to velocities[v;w] = T*dphiH

dphi=inv(T)*[v;w];
dphiH1 = dphi(1);   % driving wheels rotation rate (L)
dphiH2 = dphi(2);   % driving wheels rotation rate (R)


%% Config 5
%% Axon Kinematics
% dx, dy, dth1, dth0 -> change in position and orientation
dx = cos(th1)*cos(th1-th0)*v-cos(th1)*sin(th1-th0)*rho0*w;
dy = sin(th1)*cos(th1-th0)*v-sin(th1)*sin(th1-th0)*rho0*w;
dth1 = -sin(th1-th0)/rho1*v-(cos(th1-th0)*rho0)/rho1*w;
dth0 = w;

delthd = dth1 - dth0;

%% Trolley Kinematics
% dpsicw -> caster wheel swivel rate (change in caster wheel orientation)
dpsicw1  = -(v*(2*s_w*sin(th1-th0)*sin(psicw1-th1)-s_l*sin(th1-th0)*cos(psicw1-th1)+2* ...
    cos(th1)*cos(th1-th0)*rho1*sin(psicw1)-2*sin(th1)*cos(th1-th0)*rho1*cos(psicw1))+w*rho0*(2* ...
    s_w*cos(th1-th0)*sin(psicw1-th1)-s_l*cos(th1-th0)*cos(psicw1-th1)-2*cos(th1)*sin(th1-th0)* ...
    rho1*sin(psicw1)+2*sin(th1)*sin(th1-th0)*rho1*cos(psicw1)))/(2*dcw*rho1);

dpsicw2  = (v*(2*s_w*sin(th1-th0)*sin(psicw2-th1)+s_l*sin(th1-th0)*cos(psicw2-th1)-2* ...
    cos(th1)*cos(th1-th0)*rho1*sin(psicw2)+2*sin(th1)*cos(th1-th0)*rho1*cos(psicw2))+w*rho0*(2* ...
    s_w*cos(th1-th0)*sin(psicw2-th1)+s_l*cos(th1-th0)*cos(psicw2-th1)+2*cos(th1)*sin(th1-th0) ...
    *rho1*sin(psicw2)-2*sin(th1)*sin(th1-th0)*rho1*cos(psicw2)))/(2*dcw*rho1);

dpsicw3  = -(v*(2*s_w*sin(th1-th0)*sin(psicw3-th1)+s_l*sin(th1-th0)*cos(psicw3-th1)+2* ...
    cos(th1)*cos(th1-th0)*rho1*sin(psicw3)-2*sin(th1)*cos(th1-th0)*rho1*cos(psicw3))+w*rho0*(2* ...
    s_w*cos(th1-th0)*sin(psicw3-th1)+s_l*cos(th1-th0)*cos(psicw3-th1)-2*cos(th1)*sin(th1-th0) ...
    *rho1*sin(psicw3)+2*sin(th1)*sin(th1-th0)*rho1*cos(psicw3)))/(2*dcw*rho1);

dpsicw4  = (v*(2*s_w*sin(th1-th0)*sin(psicw4-th1)-s_l*sin(th1-th0)*cos(psicw4-th1)-2* ...
    cos(th1)*cos(th1-th0)*rho1*sin(psicw4)+2*sin(th1)*cos(th1-th0)*rho1*cos(psicw4))+w*rho0*(2* ...
    s_w*cos(th1-th0)*sin(psicw4-th1)-s_l*cos(th1-th0)*cos(psicw4-th1)+2*cos(th1)*sin(th1-th0) ...
    *rho1*sin(psicw4)-2*sin(th1)*sin(th1-th0)*rho1*cos(psicw4)))/(2*dcw*rho1);

%% Dynamics: Mpp*d?/dt + npp*? + n3p*psiCW = Bpp*?
%       ? = [v;w]; ? = [?1; ?2] 

Mpp = [[(2*IHy)/rhoH^2+(ITP*sin(th1-th0)^2)/rho1^2+mT*cos(th1-th0)^2 , (ITP*cos(th1-th0)*sin(th1-th0)*rho0)/rho1^2-mT*cos(th1-th0)*sin(th1-th0)*rho0]; ...
    [(ITP*cos(th1-th0)*sin(th1-th0)*rho0)/rho1^2-mT*cos(th1-th0)*sin(th1-th0)*rho0, (2*IHy*L^2)/rhoH^2+(ITP*cos(th1-th0)^2*rho0^2)/rho1^2+mT*sin(th1-th0)^2*rho0^2-2*e2*rho0+ITz]];

npp = [[-(delthd*cos(th1-th0)*sin(th1-th0)*(mT*rho1^2-ITP))/rho1^2, -(delthd*rho0*(mT*cos(th1-th0)^2*rho1^2+ITP*sin(th1-th0)^2)+e2*(dth0)*rho1^2-e1*(dth1)*rho0*rho1)/rho1^2];...
    [(delthd*rho0*(mT*sin(th1-th0)^2*rho1^2+ITP*cos(th1-th0)^2)+e2*(dth0)*rho1^2-e1*(dth1)*rho0*rho1)/rho1^2 , (delthd*cos(th1-th0)*sin(th1-th0)*rho0^2*(mT*rho1^2-ITP))/rho1^2]];

n3p = [[(dcw*mCW*(dpsicw1)*(s_l*sin(th1-th0)*sin(psicw1-th1)+2*cos(th1-th0)*rho1*cos(psicw1-th1)+2*s_w*sin(th1-th0)*cos(psicw1-th1)))/(2*rho1) , (dcw*mCW*(dpsicw2)*(s_l*sin(th1-th0)*sin(psicw2-th1)+2*cos(th1-th0)*rho1*cos(psicw2-th1)-2*s_w*sin(th1-th0)*cos(psicw2-th1)))/(2*rho1), ...
    -(dcw*mCW*(dpsicw3)*(s_l*sin(th1-th0)*sin(psicw3-th1)-2*s_w*sin(th1-th0)*cos(psicw3-th1)-2*sin(th1)*cos(th1-th0)*rho1*sin(psicw3)-2*cos(th1)*cos(th1-th0)*rho1*cos(psicw3)))/(2*rho1) , -(dcw*mCW*(dpsicw4)*(s_l*sin(th1-th0)*sin(psicw4-th1)+2*s_w*sin(th1-th0)*cos(psicw4-th1)-2*sin(th1)*cos(th1-th0)*rho1*sin(psicw4)-2*cos(th1)*cos(th1-th0)*rho1*cos(psicw4)))/(2*rho1)];...
    [(dcw*mCW*rho0*(dpsicw1)*(s_l*cos(th1-th0)*sin(psicw1-th1)-2*sin(th1-th0)*rho1*cos(psicw1-th1)+2*s_w*cos(th1-th0)*cos(psicw1-th1)))/(2*rho1) , (dcw*mCW*rho0*(dpsicw2)*(s_l*cos(th1-th0)*sin(psicw2-th1)-2*sin(th1-th0)*rho1*cos(psicw2-th1)-2*s_w*cos(th1-th0)*cos(psicw2-th1)))/(2*rho1), ...
    -(dcw*mCW*rho0*(dpsicw3)*(s_l*cos(th1-th0)*sin(psicw3-th1)-2*s_w*cos(th1-th0)*cos(psicw3-th1)+2*sin(th1)*sin(th1-th0)*rho1*sin(psicw3)+2*cos(th1)*sin(th1-th0)*rho1*cos(psicw3)))/(2*rho1) , -(dcw*mCW*rho0*(dpsicw4)*(s_l*cos(th1-th0)*sin(psicw4-th1)+2*s_w*cos(th1-th0)*cos(psicw4-th1)+2*sin(th1)*sin(th1-th0)*rho1*sin(psicw4)+2*cos(th1)*sin(th1-th0)*rho1*cos(psicw4)))/(2*rho1)]];

Bpp = [[1/rhoH,1/rhoH];[-L/rhoH,L/rhoH]];
tau = [tau1; tau2];

% d?/dt -> equation for the solution of the linear and angular accelerations
dvw = inv(Mpp)*(Bpp*tau - npp*[v;w] - n3p*[dpsicw1;dpsicw2;dpsicw3;dpsicw4]);
dv = dvw(1);    % linear acceleration
dw = dvw(2);    % angular acceleration

dz = [dx,dy,dth1,dth0,dpsicw1, dpsicw2, dpsicw3, dpsicw4, dv, dw].';
